simulink model "sampleModel1603"  (R2023a)
settings: Solver=VariableStepAuto  StartTime=0.0  StopTime=10.0  RelTol=1e-3
libraries: hdlsllib x7, simulink x1
settings Model: Creator=user1  LastModifiedBy=user1

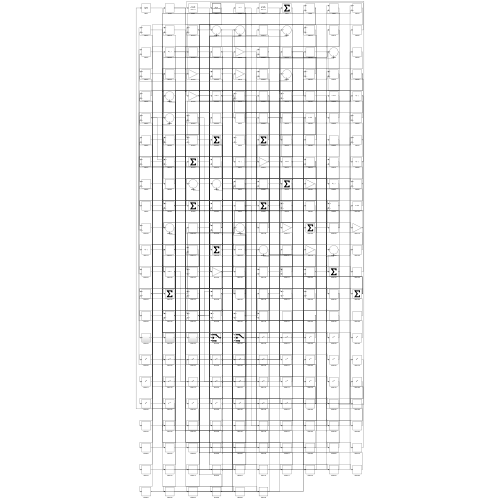
[thumbnail: Simulink's stored preview of the top-level diagram]
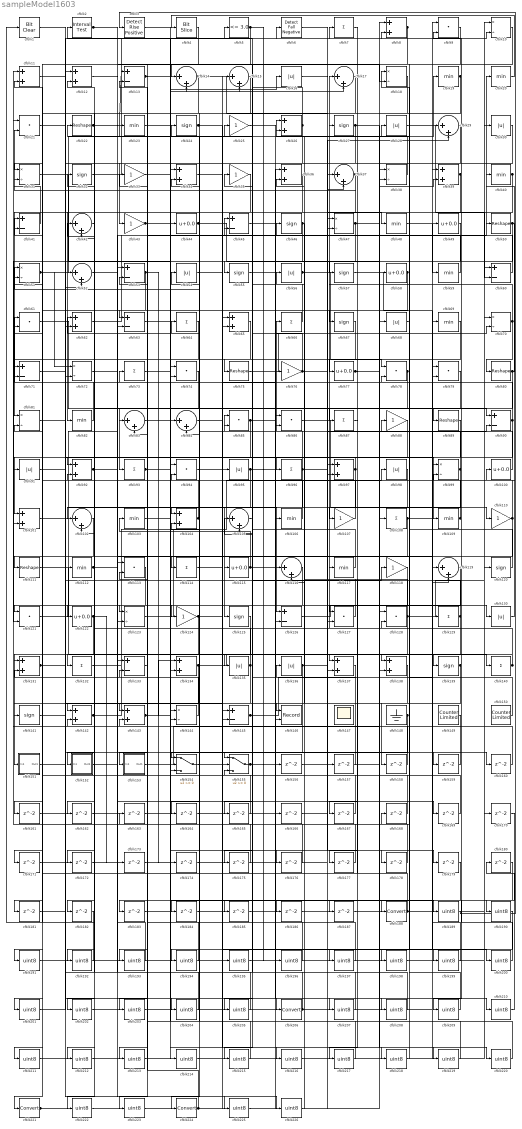
== system sampleModel1603 ==
  cfblk1 : simulink/Logic and Bit Operations/Bit Clear  iBit=0
      settings: LibrarySourceBlock=|
      | hdlsllib/Logic and Bit
      | Operations/Bit Clear
  cfblk{10,18,31,38,47,51,70,72,81,99,123,144} (12 alike) : Product  Inputs=*/  RndMeth=Zero  SaturateOnIntegerOverflow=on
  cfblk{44,49,58,77,100,115,122} (7 alike) : Bias  Bias=0.0  SaturateOnIntegerOverflow=off
  cfblk{8,11..12,26,34,36,39,62,65,92,97,101,104,131,134,137..138,142..143} (19 alike) : Sum
  cfblk{14..15,17,29,37,42,52,83..84,102,105,116,119} (13 alike) : Sum  Inputs=|++
  cfblk{19..20,23,40,48,59,69,82,103,106,109,112,117} (13 alike) : MinMax
  cfblk{25,33,35,43,76,88,107,110,118,124} (10 alike) : Gain
  cfblk{7,64,66,73,87,93,96,108,114,129,132,140} (12 alike) : Sum  Inputs=+
  cfblk{22,50,75,80,89,111} (6 alike) : Reshape
  cfblk{9,21,61,74,78..79,85..86,94,113,121,127..128} (13 alike) : DotProduct  OutDataTypeStr=Inherit: Inherit via internal rule
  cfblk{24,27,32,46,55,57,67,120,125,139,141} (11 alike) : Signum
  cfblk{13,41,45,53,60,63,71,90,126,133,145} (11 alike) : Sum  Inputs=+-
  cfblk{16,28,30,54,56,68,91,95,98,130,135..136} (12 alike) : Abs  SaturateOnIntegerOverflow=off
  cfblk146 : Record  FileSettingsInternal="{\"entries\":[{\"content\":{\"excelSettings\":{\"content\":{},\"type\":\"Streamout.ExcelSettings\"}},\"type\":\"Streamout.FileSettingStorage\",\"uuid\":\"\"}],\"packageUris\":[\"http:\\/\\/schema.mathworks.com\\/mf0\\/streamout_blocks\\/R2020a\"],\"version\":\"1.0\"}"  Layout=[1 1]  SignalsInternal="{\"entries\":[{\"content\":{\"signals\":[{\"content\":{\"blockPath\":[],\"dimensions\":[1],\"domain\":\"\",\"lineColor\":\"#a2142f\",\"plots\":[1],\"port\":1,\"signalID\":2237,\"signalName\":\"XY Graph:1\"},\"type\":\"RecordBlkView.Signal\",\"uuid\":\"\"},{\"content\":{\"blockPath\":[],\"dimensions\":[1],\"domain\":\"\",\"lineColor\":\"#139fff\",\"plots\":[1],\"port\":2,\"signalID\":2240,\"signalName\":\"XY Graph:2\"},\"type\":\"RecordBlkView.Signal\",\"uuid\":\"\"}]},\"type\":\"RecordBlkView.InputSignals\",\"uuid\":\"\"}],\"packageUris\":[\"http:\\/\\/schema.mathworks.com\\/mf0\\/streamout_blocks\\/R2020a\"],\"version\":\"1.0\"}"  VisualizationBindings="{\"xyplotplugin\":{\"info\":[{\"series\":[{\"bindingParametersList\":[{\"parameter\":\"X-Axis\",\"signalID\":2237,\"signalName\":\"XY Graph:1\"},{\"parameter\":\"Y-Axis\",\"signalID\":2240,\"signalName\":\"XY Graph:2\"}],\"seriesID\":42560}],\"subplotID\":1}]}}"  CompatibilityTag=XY  st=-1
  cfblk147 : Scope
      settings: Floating=on
  cfblk148 : Ground
  cfblk149 : hdlsllib/Sources/Counter Limited  uplimit=7  tsamp=-1
  cfblk150 : hdlsllib/Sources/Counter Limited  uplimit=7  tsamp=-1
  cfblk151 : Subsystem
      settings: LibrarySourceBlock=|
      | hdlsllib/Ports &
      | Subsystems/Subsystem
  cfblk152 : Subsystem
      settings: LibrarySourceBlock=|
      | hdlsllib/Ports &
      | Subsystems/Subsystem
  cfblk153 : Subsystem
      settings: LibrarySourceBlock=|
      | hdlsllib/Ports &
      | Subsystems/Subsystem
  cfblk154 : Switch  SaturateOnIntegerOverflow=off  InputSameDT=off
  cfblk155 : Switch  SaturateOnIntegerOverflow=off  InputSameDT=off
  cfblk{156..187} (32 alike) : Delay  SampleTime=1
  cfblk{188,206,221,224} (4 alike) : DataTypeConversion  SaturateOnIntegerOverflow=off  RndMeth=Floor
  cfblk{189..205,207..220,222..223,225..226} (35 alike) : DataTypeConversion  OutDataTypeStr=uint8  SaturateOnIntegerOverflow=off  RndMeth=Floor
  cfblk2 : hdlsllib/Logic and Bit Operations/Interval Test  IntervalClosedRight=on  uplimit=0.5  IntervalClosedLeft=on  lowlimit=-0.5  OutDataTypeStr=boolean
  cfblk3 : hdlsllib/Logic and Bit Operations/Detect Rise Positive  vinit=0  OutDataTypeStr=boolean
  cfblk4 : hdlsllib/Logic and Bit Operations/Bit Slice  lidx=7  ridx=0
  cfblk5 : hdlsllib/Logic and Bit Operations/Compare To Constant  relop=<=  const=3.0  OutDataTypeStr=boolean
  cfblk6 : hdlsllib/Logic and Bit Operations/Detect Fall Negative  vinit=0  OutDataTypeStr=boolean
  wires:
  cfblk90/1 -> cfblk51/2, cfblk165/1
  cfblk98/1 -> cfblk125/1
  cfblk56/1 -> cfblk78/1, cfblk178/1
  cfblk100/1 -> cfblk66/1
  cfblk35/1 -> cfblk81/1
  cfblk99/1 -> cfblk62/1, cfblk175/1
  cfblk62/1 -> cfblk20/1
  cfblk50/1 -> cfblk101/1, cfblk121/2
  cfblk38/1 -> cfblk26/1
  cfblk46/1 -> cfblk55/1, cfblk146/1
  cfblk124/1 -> cfblk29/1, cfblk186/1, cfblk223/1
  cfblk74/1 -> cfblk93/1
  cfblk92/1 -> cfblk53/1, cfblk99/1
  cfblk37/1 -> cfblk82/1, cfblk31/2
  cfblk115/1 -> cfblk103/1, cfblk187/1
  cfblk122/1 -> cfblk151/1(In1), cfblk172/1, cfblk173/1
  cfblk117/1 -> cfblk22/1
  cfblk51/1 -> cfblk19/1, cfblk72/1
  cfblk97/1 -> cfblk104/1, cfblk92/1
  cfblk131/1 -> cfblk154/1, cfblk159/1
  cfblk134/1 -> cfblk140/1, cfblk144/2
  cfblk10/1 -> cfblk83/1
  cfblk75/1 -> cfblk10/1
  cfblk64/1 -> cfblk142/1
  cfblk20/1 -> cfblk4/1
  cfblk132/1 -> cfblk98/1
  cfblk67/1 -> cfblk101/2
  cfblk116/1 -> cfblk224/1
  cfblk77/1 -> cfblk167/1, cfblk220/1
  cfblk18/1 -> cfblk152/1(In1)
  cfblk30/1 -> cfblk43/1
  cfblk142/1 -> cfblk44/1, cfblk42/2
  cfblk86/1 -> cfblk110/1
  cfblk140/1 -> cfblk17/1, cfblk56/1, cfblk138/1, cfblk24/1
  cfblk111/1 -> cfblk137/1
  cfblk107/1 -> cfblk53/2
  cfblk104/1 -> cfblk54/1, cfblk41/2
  cfblk103/1 -> cfblk6/1
  cfblk16/1 -> cfblk48/1
  cfblk150/1 -> cfblk88/1
  cfblk21/1 -> cfblk155/1
  cfblk17/1 -> cfblk84/2
  cfblk145/1 -> cfblk5/1, cfblk79/2
  cfblk136/1 -> cfblk90/2, cfblk164/1
  cfblk31/1 -> cfblk144/1
  cfblk4/1 -> cfblk83/2
  cfblk153/1(Out1) -> cfblk68/1
  cfblk68/1 -> cfblk18/1
  cfblk79/1 -> cfblk123/1
  cfblk137/1 -> cfblk136/1
  cfblk127/1 -> cfblk85/1
  cfblk48/1 -> cfblk59/1
  cfblk93/1 -> cfblk143/1, cfblk210/1
  cfblk130/1 -> cfblk100/1
  cfblk88/1 -> cfblk153/1(In1)
  cfblk89/1 -> cfblk109/1
  cfblk32/1 -> cfblk8/2
  cfblk70/1 -> cfblk27/1, cfblk80/1
  cfblk148/1 -> cfblk143/2, cfblk154/3
  cfblk22/1 -> cfblk13/1, cfblk119/2
  cfblk82/1 -> cfblk61/1
  cfblk44/1 -> cfblk128/1, cfblk184/1
  cfblk121/1 -> cfblk45/1
  cfblk110/1 -> cfblk42/1, cfblk181/1
  cfblk41/1 -> cfblk21/2
  cfblk57/1 -> cfblk119/1
  cfblk25/1 -> cfblk87/1
  cfblk135/1 -> cfblk132/1, cfblk92/2, cfblk141/1
  cfblk123/1 -> cfblk37/1
  cfblk13/1 -> cfblk63/1, cfblk18/2
  cfblk119/1 -> cfblk121/1
  cfblk52/1 -> cfblk139/1
  cfblk15/1 -> cfblk221/1
  cfblk143/1 -> cfblk17/2, cfblk10/2, cfblk134/1
  cfblk78/1 -> cfblk71/2, cfblk162/1
  cfblk59/1 -> cfblk33/1
  cfblk11/1 -> cfblk112/1
  cfblk26/1 -> cfblk2/1, cfblk62/2
  cfblk120/1 -> cfblk78/2
  cfblk129/1 -> cfblk25/1, cfblk135/1
  cfblk128/1 -> cfblk60/1, cfblk46/1, cfblk183/1
  cfblk2/1 -> cfblk14/1, cfblk134/2
  cfblk149/1 -> cfblk142/2
  cfblk43/1 -> cfblk115/1, cfblk16/1
  cfblk58/1 -> cfblk111/1, cfblk146/2
  cfblk27/1 -> cfblk38/2, cfblk72/2, cfblk219/1
  cfblk106/1 -> cfblk64/1
  cfblk8/1 -> cfblk31/1, cfblk215/1
  cfblk28/1 -> cfblk60/2
  cfblk96/1 -> cfblk126/1, cfblk51/1, cfblk29/2
  cfblk141/1 -> cfblk7/1
  cfblk85/1 -> cfblk36/1, cfblk91/1
  cfblk6/1 -> cfblk90/1
  cfblk19/1 -> cfblk57/1, cfblk77/1
  cfblk5/1 -> cfblk193/1, cfblk196/1
  cfblk76/1 -> cfblk97/2, cfblk45/2
  cfblk63/1 -> cfblk74/2
  cfblk95/1 -> cfblk70/2, cfblk156/1, cfblk222/1
  cfblk102/1 -> cfblk131/1
  cfblk66/1 -> cfblk35/1
  cfblk155/1 -> cfblk108/1, cfblk160/1
  cfblk61/1 -> cfblk129/1
  cfblk84/1 -> cfblk89/1
  cfblk54/1 -> cfblk50/1
  cfblk101/1 -> cfblk106/1
  cfblk1/1 -> cfblk96/1
  cfblk53/1 -> cfblk122/1, cfblk174/1
  cfblk29/1 -> cfblk67/1
  cfblk144/1 -> cfblk61/2
  cfblk12/1 -> cfblk206/1
  cfblk126/1 -> cfblk130/1
  cfblk40/1 -> cfblk71/1, cfblk107/1
  cfblk151/1(Out1) -> cfblk118/1
  cfblk39/1 -> cfblk102/1, cfblk185/1
  cfblk49/1 -> cfblk127/1
  cfblk81/1 -> cfblk145/2
  cfblk3/1 -> cfblk188/1
  cfblk112/1 -> cfblk32/1, cfblk226/1
  cfblk108/1 -> cfblk161/1, cfblk200/1
  cfblk24/1 -> cfblk114/1, cfblk179/1
  cfblk60/1 -> cfblk13/2
  cfblk139/1 -> cfblk197/1, cfblk212/1
  cfblk47/1 -> cfblk39/2, cfblk75/1
  cfblk80/1 -> cfblk124/1, cfblk40/1
  cfblk14/1 -> cfblk47/1, cfblk123/2
  cfblk109/1 -> cfblk41/1, cfblk99/2
  cfblk154/1 -> cfblk76/1
  cfblk156/1 -> cfblk36/2
  cfblk157/1 -> cfblk85/2
  cfblk138/1 -> cfblk158/1
  cfblk158/1 -> cfblk11/1
  cfblk159/1 -> cfblk26/2
  cfblk160/1 -> cfblk39/1
  cfblk161/1 -> cfblk63/2
  cfblk162/1 -> cfblk37/2
  cfblk163/1 -> cfblk84/1
  cfblk164/1 -> cfblk97/1
  cfblk165/1 -> cfblk74/1
  cfblk45/1 -> cfblk166/1
  cfblk166/1 -> cfblk137/2
  cfblk167/1 -> cfblk81/2
  cfblk168/1 -> cfblk38/1
  cfblk72/1 -> cfblk169/1
  cfblk169/1 -> cfblk155/2
  cfblk118/1 -> cfblk171/1
  cfblk171/1 -> cfblk145/1
  cfblk172/1 -> cfblk102/2
  cfblk173/1 -> cfblk126/2
  cfblk174/1 -> cfblk47/2
  cfblk175/1 -> cfblk21/1
  cfblk83/1 -> cfblk176/1
  cfblk176/1 -> cfblk104/2
  cfblk7/1 -> cfblk177/1
  cfblk177/1 -> cfblk155/3
  cfblk178/1 -> cfblk154/2
  cfblk181/1 -> cfblk52/2
  cfblk42/1 -> cfblk182/1
  cfblk182/1 -> cfblk1/1
  cfblk183/1 -> cfblk14/2
  cfblk184/1 -> cfblk127/2
  cfblk185/1 -> cfblk70/1
  cfblk186/1 -> cfblk8/1
  cfblk187/1 -> cfblk30/1
  cfblk188/1 -> cfblk28/1, cfblk117/1, cfblk131/2
  cfblk33/1 -> cfblk189/1
  cfblk189/1 -> cfblk3/1
  cfblk170/1 -> cfblk190/1
  cfblk125/1 -> cfblk191/1
  cfblk191/1 -> cfblk170/1
  cfblk113/1 -> cfblk192/1
  cfblk192/1 -> cfblk11/2
  cfblk193/1 -> cfblk113/1
  cfblk190/1 -> cfblk194/1
  cfblk194/1 -> cfblk113/2
  cfblk34/1 -> cfblk195/1
  cfblk195/1 -> cfblk105/1
  cfblk196/1 -> cfblk34/1
  cfblk197/1 -> cfblk34/2
  cfblk9/1 -> cfblk198/1
  cfblk198/1 -> cfblk79/1
  cfblk114/1 -> cfblk199/1
  cfblk199/1 -> cfblk9/1
  cfblk200/1 -> cfblk9/2
  cfblk69/1 -> cfblk201/1
  cfblk201/1 -> cfblk52/1
  cfblk36/1 -> cfblk202/1
  cfblk202/1 -> cfblk69/1
  cfblk133/1 -> cfblk203/1
  cfblk203/1 -> cfblk86/1
  cfblk91/1 -> cfblk204/1
  cfblk204/1 -> cfblk133/1
  cfblk105/1 -> cfblk205/1
  cfblk205/1 -> cfblk133/2
  cfblk206/1 -> cfblk105/2, cfblk86/2
  cfblk152/1(Out1) -> cfblk207/1
  cfblk207/1 -> cfblk12/1
  cfblk55/1 -> cfblk208/1
  cfblk208/1 -> cfblk12/2
  cfblk180/1 -> cfblk209/1
  cfblk209/1 -> cfblk128/2
  cfblk210/1 -> cfblk180/1
  cfblk65/1 -> cfblk211/1
  cfblk211/1 -> cfblk95/1
  cfblk212/1 -> cfblk65/1
  cfblk179/1 -> cfblk213/1
  cfblk213/1 -> cfblk65/2
  cfblk73/1 -> cfblk214/1
  cfblk214/1 -> cfblk49/1
  cfblk215/1 -> cfblk73/1
  cfblk23/1 -> cfblk216/1
  cfblk216/1 -> cfblk120/1
  cfblk87/1 -> cfblk217/1
  cfblk217/1 -> cfblk23/1
  cfblk94/1 -> cfblk218/1
  cfblk218/1 -> cfblk168/1
  cfblk219/1 -> cfblk94/1
  cfblk220/1 -> cfblk94/2
  cfblk221/1 -> cfblk157/1, cfblk138/2
  cfblk222/1 -> cfblk15/1
  cfblk223/1 -> cfblk15/2
  cfblk224/1 -> cfblk163/1, cfblk58/1
  cfblk71/1 -> cfblk225/1
  cfblk225/1 -> cfblk116/1
  cfblk226/1 -> cfblk116/2

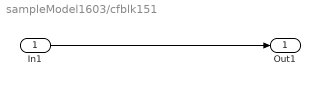
== system sampleModel1603/cfblk151 ==
  In1 : Inport
  Out1 : Outport
  wires:
  In1/1 -> Out1/1

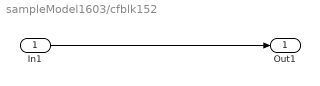
== system sampleModel1603/cfblk152 ==
  In1 : Inport
  Out1 : Outport
  wires:
  In1/1 -> Out1/1

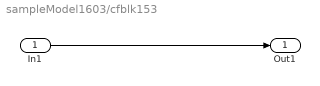
== system sampleModel1603/cfblk153 ==
  In1 : Inport
  Out1 : Outport
  wires:
  In1/1 -> Out1/1
